simulink model "Drone_Waypoint_follower"  (R2024b)
settings: Solver=VariableStepAuto  StartTime=0.0  StopTime=10.0  RelTol=1e-3
libraries: robotcorelib x1, simulink x1, uavutilslib x1, uavalgslib x1
settings Model: Creator=Adi

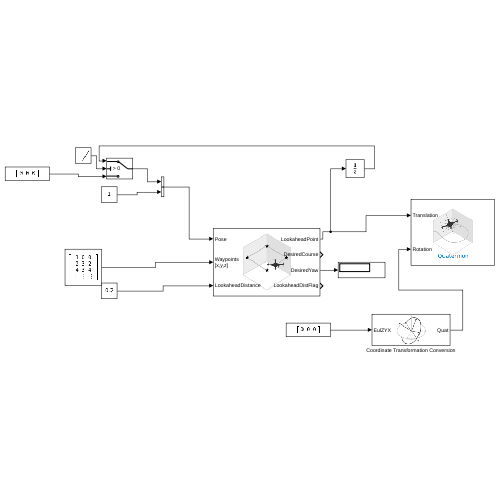
[thumbnail: Simulink's stored preview of the top-level diagram]
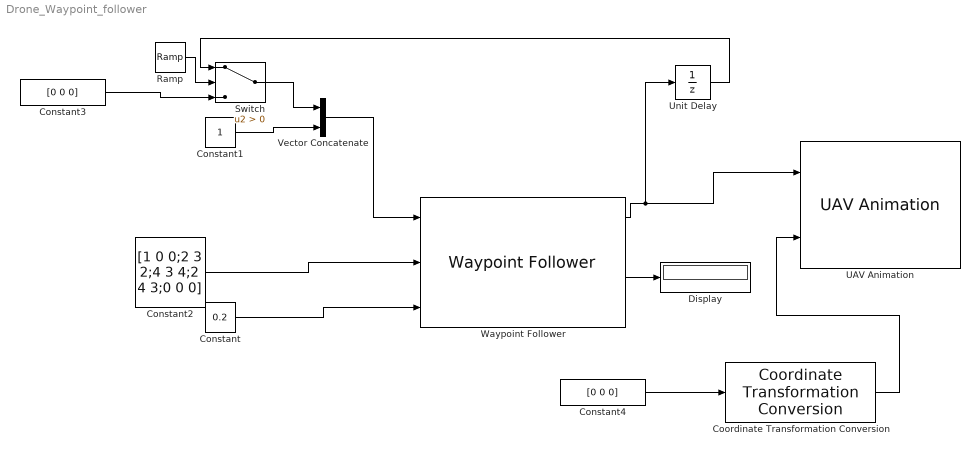
== system Drone_Waypoint_follower ==
  Constant : Constant  Value=0.2
  Constant1 : Constant
  Constant2 : Constant  Value=[1 0 0;2 3 2;4 3 4;2 4 3;0 0 0]
  Constant3 : Constant  Value=[0 0 0]
  Constant4 : Constant  Value=[0 0 0]
  Coordinate Transformation Conversion : robotcorelib/Coordinate Transformation Conversion  InputRepresentation=Euler Angles  InputEulerSequence=ZYX  ShowTrVecInputPort=on  OutputRepresentation=Quaternion  OutputEulerSequence=ZYX  ShowTrVecOutputPort=on  SimulateUsing=Interpreted execution
      settings: LibrarySourceBlock=uavutilslib/Coordinate Transformation Conversion
  Display : Display
  Ramp : simulink/Sources/Ramp  slope=1  start=0  InitialOutput=0
  Switch : Switch  Criteria=u2 > Threshold  SaturateOnIntegerOverflow=off  InputSameDT=off
  UAV Animation : uavutilslib/UAV Animation  NumUAV=1  DynamicUAVConfig=off  UAVType=Multirotor  UAVSize=1  UAVColor=[1 0 0]  UAVTrajectoryAlpha=1  InertialZDirection=Down  RotationFormat=Quaternion  DrawMarkers=off  SampleTime=-1
  Unit Delay : UnitDelay  SampleTime=-1  HasFrameUpgradeWarning=on
  Vector Concatenate : Concatenate
  Waypoint Follower : uavalgslib/Waypoint Follower  UAVType=multirotor  StartFrom=first  TransitionRadiusSource=internal  TransitionRadius=10  MinLookaheadDistance=0.1  HoverAtLastWaypoint=off  YawInput=off  ShowCrossTrackErrorOutput=off  ShowStatusOutput=off  SimulateUsing=Interpreted execution
  wires:
  Coordinate Transformation Conversion/1 -> UAV Animation/2
  Constant/1 -> Waypoint Follower/3
  Waypoint Follower/1 -> Unit Delay/1, UAV Animation/1
  Constant1/1 -> Vector Concatenate/2
  Switch/1 -> Vector Concatenate/1
  Ramp/1 -> Switch/2
  Constant3/1 -> Switch/3
  Constant4/1 -> Coordinate Transformation Conversion/1
  Unit Delay/1 -> Switch/1
  Vector Concatenate/1 -> Waypoint Follower/1
  Waypoint Follower/3 -> Display/1
  Constant2/1 -> Waypoint Follower/2
